simulink model "microarchi_router"  (R2015a)
settings: Solver=ode45  StartTime=0.0  StopTime=10.0  RelTol=1e-3
undefined symbols (not defined in the file or in its folder): des
(part 2 of 2)

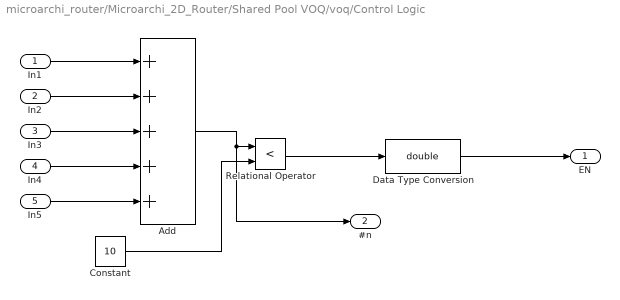
== system microarchi_router/Microarchi_2D_Router/Shared Pool VOQ/voq/Control Logic ==
  In1 : Inport
  In2 : Inport  Port=2
  In3 : Inport  Port=3
  In4 : Inport  Port=4
  In5 : Inport  Port=5
  Add : Sum  Inputs=+++++
  Constant : Constant  Value=10
  Data Type Conversion : DataTypeConversion  OutDataTypeStr=double
  Relational Operator : RelationalOperator  Operator=<
  EN : Outport  OutDataTypeStr=double
  #n : Outport  Port=2
  wires:
  In1/1 -> Add/1
  In2/1 -> Add/2
  In3/1 -> Add/3
  Constant/1 -> Relational Operator/2
  Add/1 -> #n/1, Relational Operator/1
  Relational Operator/1 -> Data Type Conversion/1
  Data Type Conversion/1 -> EN/1
  In4/1 -> Add/4
  In5/1 -> Add/5

== system microarchi_router/Microarchi_2D_Router/Shared Pool VOQ/voq/Release1 ==
  EN : Inport
  CLK : Inport  Port=2
  Enabled Gate6 : EnabledGate
  Out : PMIOPort  Port=1  Side=Right
  In : PMIOPort  Port=2  Side=Left
  wires:
  CLK/1 -> ?
  EN/1 -> Enabled Gate6/1
  connections:
  In/RConn1 -- Enabled Gate6/LConn1
  Enabled Gate6/RConn1 -- Out/RConn1

== system microarchi_router/Microarchi_2D_Router/Shared Pool VOQ/voq/Release2 ==
  EN : Inport
  CLK : Inport  Port=2
  Enabled Gate6 : EnabledGate
  Out : PMIOPort  Port=1  Side=Right
  In : PMIOPort  Port=2  Side=Left
  wires:
  EN/1 -> Enabled Gate6/1
  CLK/1 -> ?
  connections:
  Enabled Gate6/RConn1 -- Out/RConn1
  In/RConn1 -- Enabled Gate6/LConn1

== system microarchi_router/Microarchi_2D_Router/Shared Pool VOQ/voq/Release3 ==
  EN : Inport
  CLK : Inport  Port=2
  Enabled Gate6 : EnabledGate
  Out : PMIOPort  Port=1  Side=Right
  In : PMIOPort  Port=2  Side=Left
  wires:
  CLK/1 -> ?
  EN/1 -> Enabled Gate6/1
  connections:
  In/RConn1 -- Enabled Gate6/LConn1
  Enabled Gate6/RConn1 -- Out/RConn1

== system microarchi_router/Microarchi_2D_Router/Shared Pool VOQ/voq/Release4 ==
  EN : Inport
  CLK : Inport  Port=2
  Enabled Gate6 : EnabledGate
  Out : PMIOPort  Port=1  Side=Right
  In : PMIOPort  Port=2  Side=Left
  wires:
  EN/1 -> Enabled Gate6/1
  CLK/1 -> ?
  connections:
  Enabled Gate6/RConn1 -- Out/RConn1
  In/RConn1 -- Enabled Gate6/LConn1

== system microarchi_router/Microarchi_2D_Router/Shared Pool VOQ/voq/Release5 ==
  EN : Inport
  CLK : Inport  Port=2
  Enabled Gate6 : EnabledGate
  Out : PMIOPort  Port=1  Side=Right
  In : PMIOPort  Port=2  Side=Left
  wires:
  CLK/1 -> ?
  EN/1 -> Enabled Gate6/1
  connections:
  In/RConn1 -- Enabled Gate6/LConn1
  Enabled Gate6/RConn1 -- Out/RConn1

== system microarchi_router/Microarchi_2D_Router/Shared Pool VOQ1/voq/Clocked FIFO1 ==
  CLK : Inport
  FIFO Queue : FIFOQueue  Capacity=F  StatNumberInBlock=on
      settings: OutputPortMap=o1
  Release Gate : ReleaseGate  OpenGateUpon=Function call from port fcn
  Single Server : SingleServer  ServiceTime=0
  Input : PMIOPort  Port=1  Side=Left
  Output : PMIOPort  Port=2  Side=Right
  #n : Outport
  wires:
  CLK/1 -> Release Gate/1
  FIFO Queue/1 -> #n/1
  connections:
  FIFO Queue/LConn1 -- Input/RConn1
  Release Gate/RConn1 -- Output/RConn1
  Single Server/RConn1 -- Release Gate/LConn1
  FIFO Queue/RConn1 -- Single Server/LConn1

== system microarchi_router/Microarchi_2D_Router/Shared Pool VOQ1/voq/Clocked FIFO2 ==
  CLK : Inport
  FIFO Queue : FIFOQueue  Capacity=F  StatNumberInBlock=on
      settings: OutputPortMap=o1
  Release Gate : ReleaseGate  OpenGateUpon=Function call from port fcn
  Single Server : SingleServer  ServiceTime=0
  Input : PMIOPort  Port=1  Side=Left
  Output : PMIOPort  Port=2  Side=Right
  #n : Outport
  wires:
  FIFO Queue/1 -> #n/1
  CLK/1 -> Release Gate/1
  connections:
  FIFO Queue/RConn1 -- Single Server/LConn1
  Single Server/RConn1 -- Release Gate/LConn1
  Release Gate/RConn1 -- Output/RConn1
  FIFO Queue/LConn1 -- Input/RConn1

== system microarchi_router/Microarchi_2D_Router/Shared Pool VOQ1/voq/Clocked FIFO3 ==
  CLK : Inport
  FIFO Queue : FIFOQueue  Capacity=F  StatNumberInBlock=on
      settings: OutputPortMap=o1
  Release Gate : ReleaseGate  OpenGateUpon=Function call from port fcn
  Single Server : SingleServer  ServiceTime=0
  Input : PMIOPort  Port=1  Side=Left
  Output : PMIOPort  Port=2  Side=Right
  #n : Outport
  wires:
  CLK/1 -> Release Gate/1
  FIFO Queue/1 -> #n/1
  connections:
  FIFO Queue/LConn1 -- Input/RConn1
  Release Gate/RConn1 -- Output/RConn1
  Single Server/RConn1 -- Release Gate/LConn1
  FIFO Queue/RConn1 -- Single Server/LConn1

== system microarchi_router/Microarchi_2D_Router/Shared Pool VOQ1/voq/Clocked FIFO4 ==
  CLK : Inport
  FIFO Queue : FIFOQueue  Capacity=F  StatNumberInBlock=on
      settings: OutputPortMap=o1
  Release Gate : ReleaseGate  OpenGateUpon=Function call from port fcn
  Single Server : SingleServer  ServiceTime=0
  Input : PMIOPort  Port=1  Side=Left
  Output : PMIOPort  Port=2  Side=Right
  #n : Outport
  wires:
  FIFO Queue/1 -> #n/1
  CLK/1 -> Release Gate/1
  connections:
  FIFO Queue/RConn1 -- Single Server/LConn1
  Single Server/RConn1 -- Release Gate/LConn1
  Release Gate/RConn1 -- Output/RConn1
  FIFO Queue/LConn1 -- Input/RConn1

== system microarchi_router/Microarchi_2D_Router/Shared Pool VOQ1/voq/Clocked FIFO5 ==
  CLK : Inport
  FIFO Queue : FIFOQueue  Capacity=F  StatNumberInBlock=on
      settings: OutputPortMap=o1
  Release Gate : ReleaseGate  OpenGateUpon=Function call from port fcn
  Single Server : SingleServer  ServiceTime=0
  Input : PMIOPort  Port=1  Side=Left
  Output : PMIOPort  Port=2  Side=Right
  #n : Outport
  wires:
  CLK/1 -> Release Gate/1
  FIFO Queue/1 -> #n/1
  connections:
  FIFO Queue/LConn1 -- Input/RConn1
  Release Gate/RConn1 -- Output/RConn1
  Single Server/RConn1 -- Release Gate/LConn1
  FIFO Queue/RConn1 -- Single Server/LConn1

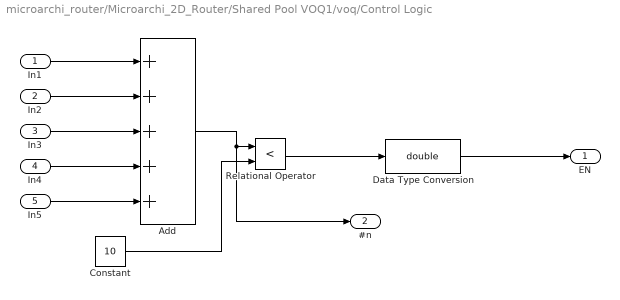
== system microarchi_router/Microarchi_2D_Router/Shared Pool VOQ1/voq/Control Logic ==
  In1 : Inport
  In2 : Inport  Port=2
  In3 : Inport  Port=3
  In4 : Inport  Port=4
  In5 : Inport  Port=5
  Add : Sum  Inputs=+++++
  Constant : Constant  Value=10
  Data Type Conversion : DataTypeConversion  OutDataTypeStr=double
  Relational Operator : RelationalOperator  Operator=<
  EN : Outport  OutDataTypeStr=double
  #n : Outport  Port=2
  wires:
  In5/1 -> Add/5
  In4/1 -> Add/4
  Data Type Conversion/1 -> EN/1
  Relational Operator/1 -> Data Type Conversion/1
  Add/1 -> Relational Operator/1, #n/1
  Constant/1 -> Relational Operator/2
  In3/1 -> Add/3
  In2/1 -> Add/2
  In1/1 -> Add/1

== system microarchi_router/Microarchi_2D_Router/Shared Pool VOQ1/voq/Release1 ==
  EN : Inport
  CLK : Inport  Port=2
  Enabled Gate6 : EnabledGate
  Out : PMIOPort  Port=1  Side=Right
  In : PMIOPort  Port=2  Side=Left
  wires:
  EN/1 -> Enabled Gate6/1
  CLK/1 -> ?
  connections:
  Enabled Gate6/RConn1 -- Out/RConn1
  In/RConn1 -- Enabled Gate6/LConn1

== system microarchi_router/Microarchi_2D_Router/Shared Pool VOQ1/voq/Release2 ==
  EN : Inport
  CLK : Inport  Port=2
  Enabled Gate6 : EnabledGate
  Out : PMIOPort  Port=1  Side=Right
  In : PMIOPort  Port=2  Side=Left
  wires:
  CLK/1 -> ?
  EN/1 -> Enabled Gate6/1
  connections:
  In/RConn1 -- Enabled Gate6/LConn1
  Enabled Gate6/RConn1 -- Out/RConn1

== system microarchi_router/Microarchi_2D_Router/Shared Pool VOQ1/voq/Release3 ==
  EN : Inport
  CLK : Inport  Port=2
  Enabled Gate6 : EnabledGate
  Out : PMIOPort  Port=1  Side=Right
  In : PMIOPort  Port=2  Side=Left
  wires:
  EN/1 -> Enabled Gate6/1
  CLK/1 -> ?
  connections:
  Enabled Gate6/RConn1 -- Out/RConn1
  In/RConn1 -- Enabled Gate6/LConn1

== system microarchi_router/Microarchi_2D_Router/Shared Pool VOQ1/voq/Release4 ==
  EN : Inport
  CLK : Inport  Port=2
  Enabled Gate6 : EnabledGate
  Out : PMIOPort  Port=1  Side=Right
  In : PMIOPort  Port=2  Side=Left
  wires:
  CLK/1 -> ?
  EN/1 -> Enabled Gate6/1
  connections:
  In/RConn1 -- Enabled Gate6/LConn1
  Enabled Gate6/RConn1 -- Out/RConn1

== system microarchi_router/Microarchi_2D_Router/Shared Pool VOQ1/voq/Release5 ==
  EN : Inport
  CLK : Inport  Port=2
  Enabled Gate6 : EnabledGate
  Out : PMIOPort  Port=1  Side=Right
  In : PMIOPort  Port=2  Side=Left
  wires:
  EN/1 -> Enabled Gate6/1
  CLK/1 -> ?
  connections:
  Enabled Gate6/RConn1 -- Out/RConn1
  In/RConn1 -- Enabled Gate6/LConn1

== system microarchi_router/Microarchi_2D_Router/Shared Pool VOQ2/voq/Clocked FIFO1 ==
  CLK : Inport
  FIFO Queue : FIFOQueue  Capacity=F  StatNumberInBlock=on
      settings: OutputPortMap=o1
  Release Gate : ReleaseGate  OpenGateUpon=Function call from port fcn
  Single Server : SingleServer  ServiceTime=0
  Input : PMIOPort  Port=1  Side=Left
  Output : PMIOPort  Port=2  Side=Right
  #n : Outport
  wires:
  FIFO Queue/1 -> #n/1
  CLK/1 -> Release Gate/1
  connections:
  FIFO Queue/RConn1 -- Single Server/LConn1
  Single Server/RConn1 -- Release Gate/LConn1
  Release Gate/RConn1 -- Output/RConn1
  FIFO Queue/LConn1 -- Input/RConn1

== system microarchi_router/Microarchi_2D_Router/Shared Pool VOQ2/voq/Clocked FIFO2 ==
  CLK : Inport
  FIFO Queue : FIFOQueue  Capacity=F  StatNumberInBlock=on
      settings: OutputPortMap=o1
  Release Gate : ReleaseGate  OpenGateUpon=Function call from port fcn
  Single Server : SingleServer  ServiceTime=0
  Input : PMIOPort  Port=1  Side=Left
  Output : PMIOPort  Port=2  Side=Right
  #n : Outport
  wires:
  CLK/1 -> Release Gate/1
  FIFO Queue/1 -> #n/1
  connections:
  FIFO Queue/LConn1 -- Input/RConn1
  Release Gate/RConn1 -- Output/RConn1
  Single Server/RConn1 -- Release Gate/LConn1
  FIFO Queue/RConn1 -- Single Server/LConn1

== system microarchi_router/Microarchi_2D_Router/Shared Pool VOQ2/voq/Clocked FIFO3 ==
  CLK : Inport
  FIFO Queue : FIFOQueue  Capacity=F  StatNumberInBlock=on
      settings: OutputPortMap=o1
  Release Gate : ReleaseGate  OpenGateUpon=Function call from port fcn
  Single Server : SingleServer  ServiceTime=0
  Input : PMIOPort  Port=1  Side=Left
  Output : PMIOPort  Port=2  Side=Right
  #n : Outport
  wires:
  FIFO Queue/1 -> #n/1
  CLK/1 -> Release Gate/1
  connections:
  FIFO Queue/RConn1 -- Single Server/LConn1
  Single Server/RConn1 -- Release Gate/LConn1
  Release Gate/RConn1 -- Output/RConn1
  FIFO Queue/LConn1 -- Input/RConn1

== system microarchi_router/Microarchi_2D_Router/Shared Pool VOQ2/voq/Clocked FIFO4 ==
  CLK : Inport
  FIFO Queue : FIFOQueue  Capacity=F  StatNumberInBlock=on
      settings: OutputPortMap=o1
  Release Gate : ReleaseGate  OpenGateUpon=Function call from port fcn
  Single Server : SingleServer  ServiceTime=0
  Input : PMIOPort  Port=1  Side=Left
  Output : PMIOPort  Port=2  Side=Right
  #n : Outport
  wires:
  CLK/1 -> Release Gate/1
  FIFO Queue/1 -> #n/1
  connections:
  FIFO Queue/LConn1 -- Input/RConn1
  Release Gate/RConn1 -- Output/RConn1
  Single Server/RConn1 -- Release Gate/LConn1
  FIFO Queue/RConn1 -- Single Server/LConn1

== system microarchi_router/Microarchi_2D_Router/Shared Pool VOQ2/voq/Clocked FIFO5 ==
  CLK : Inport
  FIFO Queue : FIFOQueue  Capacity=F  StatNumberInBlock=on
      settings: OutputPortMap=o1
  Release Gate : ReleaseGate  OpenGateUpon=Function call from port fcn
  Single Server : SingleServer  ServiceTime=0
  Input : PMIOPort  Port=1  Side=Left
  Output : PMIOPort  Port=2  Side=Right
  #n : Outport
  wires:
  FIFO Queue/1 -> #n/1
  CLK/1 -> Release Gate/1
  connections:
  FIFO Queue/RConn1 -- Single Server/LConn1
  Single Server/RConn1 -- Release Gate/LConn1
  Release Gate/RConn1 -- Output/RConn1
  FIFO Queue/LConn1 -- Input/RConn1

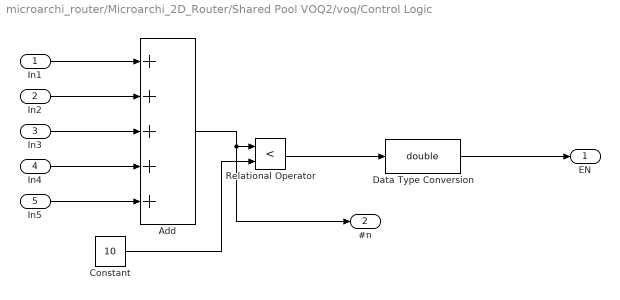
== system microarchi_router/Microarchi_2D_Router/Shared Pool VOQ2/voq/Control Logic ==
  In1 : Inport
  In2 : Inport  Port=2
  In3 : Inport  Port=3
  In4 : Inport  Port=4
  In5 : Inport  Port=5
  Add : Sum  Inputs=+++++
  Constant : Constant  Value=10
  Data Type Conversion : DataTypeConversion  OutDataTypeStr=double
  Relational Operator : RelationalOperator  Operator=<
  EN : Outport  OutDataTypeStr=double
  #n : Outport  Port=2
  wires:
  In1/1 -> Add/1
  In2/1 -> Add/2
  In3/1 -> Add/3
  Constant/1 -> Relational Operator/2
  Add/1 -> #n/1, Relational Operator/1
  Relational Operator/1 -> Data Type Conversion/1
  Data Type Conversion/1 -> EN/1
  In4/1 -> Add/4
  In5/1 -> Add/5

== system microarchi_router/Microarchi_2D_Router/Shared Pool VOQ2/voq/Release1 ==
  EN : Inport
  CLK : Inport  Port=2
  Enabled Gate6 : EnabledGate
  Out : PMIOPort  Port=1  Side=Right
  In : PMIOPort  Port=2  Side=Left
  wires:
  CLK/1 -> ?
  EN/1 -> Enabled Gate6/1
  connections:
  In/RConn1 -- Enabled Gate6/LConn1
  Enabled Gate6/RConn1 -- Out/RConn1

== system microarchi_router/Microarchi_2D_Router/Shared Pool VOQ2/voq/Release2 ==
  EN : Inport
  CLK : Inport  Port=2
  Enabled Gate6 : EnabledGate
  Out : PMIOPort  Port=1  Side=Right
  In : PMIOPort  Port=2  Side=Left
  wires:
  EN/1 -> Enabled Gate6/1
  CLK/1 -> ?
  connections:
  Enabled Gate6/RConn1 -- Out/RConn1
  In/RConn1 -- Enabled Gate6/LConn1

== system microarchi_router/Microarchi_2D_Router/Shared Pool VOQ2/voq/Release3 ==
  EN : Inport
  CLK : Inport  Port=2
  Enabled Gate6 : EnabledGate
  Out : PMIOPort  Port=1  Side=Right
  In : PMIOPort  Port=2  Side=Left
  wires:
  CLK/1 -> ?
  EN/1 -> Enabled Gate6/1
  connections:
  In/RConn1 -- Enabled Gate6/LConn1
  Enabled Gate6/RConn1 -- Out/RConn1

== system microarchi_router/Microarchi_2D_Router/Shared Pool VOQ2/voq/Release4 ==
  EN : Inport
  CLK : Inport  Port=2
  Enabled Gate6 : EnabledGate
  Out : PMIOPort  Port=1  Side=Right
  In : PMIOPort  Port=2  Side=Left
  wires:
  EN/1 -> Enabled Gate6/1
  CLK/1 -> ?
  connections:
  Enabled Gate6/RConn1 -- Out/RConn1
  In/RConn1 -- Enabled Gate6/LConn1

== system microarchi_router/Microarchi_2D_Router/Shared Pool VOQ2/voq/Release5 ==
  EN : Inport
  CLK : Inport  Port=2
  Enabled Gate6 : EnabledGate
  Out : PMIOPort  Port=1  Side=Right
  In : PMIOPort  Port=2  Side=Left
  wires:
  CLK/1 -> ?
  EN/1 -> Enabled Gate6/1
  connections:
  In/RConn1 -- Enabled Gate6/LConn1
  Enabled Gate6/RConn1 -- Out/RConn1

== system microarchi_router/Microarchi_2D_Router/Shared Pool VOQ3/voq/Clocked FIFO1 ==
  CLK : Inport
  FIFO Queue : FIFOQueue  Capacity=F  StatNumberInBlock=on
      settings: OutputPortMap=o1
  Release Gate : ReleaseGate  OpenGateUpon=Function call from port fcn
  Single Server : SingleServer  ServiceTime=0
  Input : PMIOPort  Port=1  Side=Left
  Output : PMIOPort  Port=2  Side=Right
  #n : Outport
  wires:
  CLK/1 -> Release Gate/1
  FIFO Queue/1 -> #n/1
  connections:
  FIFO Queue/LConn1 -- Input/RConn1
  Release Gate/RConn1 -- Output/RConn1
  Single Server/RConn1 -- Release Gate/LConn1
  FIFO Queue/RConn1 -- Single Server/LConn1

== system microarchi_router/Microarchi_2D_Router/Shared Pool VOQ3/voq/Clocked FIFO2 ==
  CLK : Inport
  FIFO Queue : FIFOQueue  Capacity=F  StatNumberInBlock=on
      settings: OutputPortMap=o1
  Release Gate : ReleaseGate  OpenGateUpon=Function call from port fcn
  Single Server : SingleServer  ServiceTime=0
  Input : PMIOPort  Port=1  Side=Left
  Output : PMIOPort  Port=2  Side=Right
  #n : Outport
  wires:
  FIFO Queue/1 -> #n/1
  CLK/1 -> Release Gate/1
  connections:
  FIFO Queue/RConn1 -- Single Server/LConn1
  Single Server/RConn1 -- Release Gate/LConn1
  Release Gate/RConn1 -- Output/RConn1
  FIFO Queue/LConn1 -- Input/RConn1

== system microarchi_router/Microarchi_2D_Router/Shared Pool VOQ3/voq/Clocked FIFO3 ==
  CLK : Inport
  FIFO Queue : FIFOQueue  Capacity=F  StatNumberInBlock=on
      settings: OutputPortMap=o1
  Release Gate : ReleaseGate  OpenGateUpon=Function call from port fcn
  Single Server : SingleServer  ServiceTime=0
  Input : PMIOPort  Port=1  Side=Left
  Output : PMIOPort  Port=2  Side=Right
  #n : Outport
  wires:
  CLK/1 -> Release Gate/1
  FIFO Queue/1 -> #n/1
  connections:
  FIFO Queue/LConn1 -- Input/RConn1
  Release Gate/RConn1 -- Output/RConn1
  Single Server/RConn1 -- Release Gate/LConn1
  FIFO Queue/RConn1 -- Single Server/LConn1

== system microarchi_router/Microarchi_2D_Router/Shared Pool VOQ3/voq/Clocked FIFO4 ==
  CLK : Inport
  FIFO Queue : FIFOQueue  Capacity=F  StatNumberInBlock=on
      settings: OutputPortMap=o1
  Release Gate : ReleaseGate  OpenGateUpon=Function call from port fcn
  Single Server : SingleServer  ServiceTime=0
  Input : PMIOPort  Port=1  Side=Left
  Output : PMIOPort  Port=2  Side=Right
  #n : Outport
  wires:
  FIFO Queue/1 -> #n/1
  CLK/1 -> Release Gate/1
  connections:
  FIFO Queue/RConn1 -- Single Server/LConn1
  Single Server/RConn1 -- Release Gate/LConn1
  Release Gate/RConn1 -- Output/RConn1
  FIFO Queue/LConn1 -- Input/RConn1

== system microarchi_router/Microarchi_2D_Router/Shared Pool VOQ3/voq/Clocked FIFO5 ==
  CLK : Inport
  FIFO Queue : FIFOQueue  Capacity=F  StatNumberInBlock=on
      settings: OutputPortMap=o1
  Release Gate : ReleaseGate  OpenGateUpon=Function call from port fcn
  Single Server : SingleServer  ServiceTime=0
  Input : PMIOPort  Port=1  Side=Left
  Output : PMIOPort  Port=2  Side=Right
  #n : Outport
  wires:
  CLK/1 -> Release Gate/1
  FIFO Queue/1 -> #n/1
  connections:
  FIFO Queue/LConn1 -- Input/RConn1
  Release Gate/RConn1 -- Output/RConn1
  Single Server/RConn1 -- Release Gate/LConn1
  FIFO Queue/RConn1 -- Single Server/LConn1

== system microarchi_router/Microarchi_2D_Router/Shared Pool VOQ3/voq/Control Logic ==
  In1 : Inport
  In2 : Inport  Port=2
  In3 : Inport  Port=3
  In4 : Inport  Port=4
  In5 : Inport  Port=5
  Add : Sum  Inputs=+++++
  Constant : Constant  Value=10
  Data Type Conversion : DataTypeConversion  OutDataTypeStr=double
  Relational Operator : RelationalOperator  Operator=<
  EN : Outport  OutDataTypeStr=double
  #n : Outport  Port=2
  wires:
  In5/1 -> Add/5
  In4/1 -> Add/4
  Data Type Conversion/1 -> EN/1
  Relational Operator/1 -> Data Type Conversion/1
  Add/1 -> Relational Operator/1, #n/1
  Constant/1 -> Relational Operator/2
  In3/1 -> Add/3
  In2/1 -> Add/2
  In1/1 -> Add/1

== system microarchi_router/Microarchi_2D_Router/Shared Pool VOQ3/voq/Release1 ==
  EN : Inport
  CLK : Inport  Port=2
  Enabled Gate6 : EnabledGate
  Out : PMIOPort  Port=1  Side=Right
  In : PMIOPort  Port=2  Side=Left
  wires:
  EN/1 -> Enabled Gate6/1
  CLK/1 -> ?
  connections:
  Enabled Gate6/RConn1 -- Out/RConn1
  In/RConn1 -- Enabled Gate6/LConn1

== system microarchi_router/Microarchi_2D_Router/Shared Pool VOQ3/voq/Release2 ==
  EN : Inport
  CLK : Inport  Port=2
  Enabled Gate6 : EnabledGate
  Out : PMIOPort  Port=1  Side=Right
  In : PMIOPort  Port=2  Side=Left
  wires:
  CLK/1 -> ?
  EN/1 -> Enabled Gate6/1
  connections:
  In/RConn1 -- Enabled Gate6/LConn1
  Enabled Gate6/RConn1 -- Out/RConn1

== system microarchi_router/Microarchi_2D_Router/Shared Pool VOQ3/voq/Release3 ==
  EN : Inport
  CLK : Inport  Port=2
  Enabled Gate6 : EnabledGate
  Out : PMIOPort  Port=1  Side=Right
  In : PMIOPort  Port=2  Side=Left
  wires:
  EN/1 -> Enabled Gate6/1
  CLK/1 -> ?
  connections:
  Enabled Gate6/RConn1 -- Out/RConn1
  In/RConn1 -- Enabled Gate6/LConn1

== system microarchi_router/Microarchi_2D_Router/Shared Pool VOQ3/voq/Release4 ==
  EN : Inport
  CLK : Inport  Port=2
  Enabled Gate6 : EnabledGate
  Out : PMIOPort  Port=1  Side=Right
  In : PMIOPort  Port=2  Side=Left
  wires:
  CLK/1 -> ?
  EN/1 -> Enabled Gate6/1
  connections:
  In/RConn1 -- Enabled Gate6/LConn1
  Enabled Gate6/RConn1 -- Out/RConn1

== system microarchi_router/Microarchi_2D_Router/Shared Pool VOQ3/voq/Release5 ==
  EN : Inport
  CLK : Inport  Port=2
  Enabled Gate6 : EnabledGate
  Out : PMIOPort  Port=1  Side=Right
  In : PMIOPort  Port=2  Side=Left
  wires:
  EN/1 -> Enabled Gate6/1
  CLK/1 -> ?
  connections:
  Enabled Gate6/RConn1 -- Out/RConn1
  In/RConn1 -- Enabled Gate6/LConn1

== system microarchi_router/Microarchi_2D_Router/Shared Pool VOQ4/voq/Clocked FIFO1 ==
  CLK : Inport
  FIFO Queue : FIFOQueue  Capacity=F  StatNumberInBlock=on
      settings: OutputPortMap=o1
  Release Gate : ReleaseGate  OpenGateUpon=Function call from port fcn
  Single Server : SingleServer  ServiceTime=0
  Input : PMIOPort  Port=1  Side=Left
  Output : PMIOPort  Port=2  Side=Right
  #n : Outport
  wires:
  FIFO Queue/1 -> #n/1
  CLK/1 -> Release Gate/1
  connections:
  FIFO Queue/RConn1 -- Single Server/LConn1
  Single Server/RConn1 -- Release Gate/LConn1
  Release Gate/RConn1 -- Output/RConn1
  FIFO Queue/LConn1 -- Input/RConn1

== system microarchi_router/Microarchi_2D_Router/Shared Pool VOQ4/voq/Clocked FIFO2 ==
  CLK : Inport
  FIFO Queue : FIFOQueue  Capacity=F  StatNumberInBlock=on
      settings: OutputPortMap=o1
  Release Gate : ReleaseGate  OpenGateUpon=Function call from port fcn
  Single Server : SingleServer  ServiceTime=0
  Input : PMIOPort  Port=1  Side=Left
  Output : PMIOPort  Port=2  Side=Right
  #n : Outport
  wires:
  CLK/1 -> Release Gate/1
  FIFO Queue/1 -> #n/1
  connections:
  FIFO Queue/LConn1 -- Input/RConn1
  Release Gate/RConn1 -- Output/RConn1
  Single Server/RConn1 -- Release Gate/LConn1
  FIFO Queue/RConn1 -- Single Server/LConn1

== system microarchi_router/Microarchi_2D_Router/Shared Pool VOQ4/voq/Clocked FIFO3 ==
  CLK : Inport
  FIFO Queue : FIFOQueue  Capacity=F  StatNumberInBlock=on
      settings: OutputPortMap=o1
  Release Gate : ReleaseGate  OpenGateUpon=Function call from port fcn
  Single Server : SingleServer  ServiceTime=0
  Input : PMIOPort  Port=1  Side=Left
  Output : PMIOPort  Port=2  Side=Right
  #n : Outport
  wires:
  FIFO Queue/1 -> #n/1
  CLK/1 -> Release Gate/1
  connections:
  FIFO Queue/RConn1 -- Single Server/LConn1
  Single Server/RConn1 -- Release Gate/LConn1
  Release Gate/RConn1 -- Output/RConn1
  FIFO Queue/LConn1 -- Input/RConn1

== system microarchi_router/Microarchi_2D_Router/Shared Pool VOQ4/voq/Clocked FIFO4 ==
  CLK : Inport
  FIFO Queue : FIFOQueue  Capacity=F  StatNumberInBlock=on
      settings: OutputPortMap=o1
  Release Gate : ReleaseGate  OpenGateUpon=Function call from port fcn
  Single Server : SingleServer  ServiceTime=0
  Input : PMIOPort  Port=1  Side=Left
  Output : PMIOPort  Port=2  Side=Right
  #n : Outport
  wires:
  CLK/1 -> Release Gate/1
  FIFO Queue/1 -> #n/1
  connections:
  FIFO Queue/LConn1 -- Input/RConn1
  Release Gate/RConn1 -- Output/RConn1
  Single Server/RConn1 -- Release Gate/LConn1
  FIFO Queue/RConn1 -- Single Server/LConn1

== system microarchi_router/Microarchi_2D_Router/Shared Pool VOQ4/voq/Clocked FIFO5 ==
  CLK : Inport
  FIFO Queue : FIFOQueue  Capacity=F  StatNumberInBlock=on
      settings: OutputPortMap=o1
  Release Gate : ReleaseGate  OpenGateUpon=Function call from port fcn
  Single Server : SingleServer  ServiceTime=0
  Input : PMIOPort  Port=1  Side=Left
  Output : PMIOPort  Port=2  Side=Right
  #n : Outport
  wires:
  FIFO Queue/1 -> #n/1
  CLK/1 -> Release Gate/1
  connections:
  FIFO Queue/RConn1 -- Single Server/LConn1
  Single Server/RConn1 -- Release Gate/LConn1
  Release Gate/RConn1 -- Output/RConn1
  FIFO Queue/LConn1 -- Input/RConn1

== system microarchi_router/Microarchi_2D_Router/Shared Pool VOQ4/voq/Control Logic ==
  In1 : Inport
  In2 : Inport  Port=2
  In3 : Inport  Port=3
  In4 : Inport  Port=4
  In5 : Inport  Port=5
  Add : Sum  Inputs=+++++
  Constant : Constant  Value=10
  Data Type Conversion : DataTypeConversion  OutDataTypeStr=double
  Relational Operator : RelationalOperator  Operator=<
  EN : Outport  OutDataTypeStr=double
  #n : Outport  Port=2
  wires:
  In1/1 -> Add/1
  In2/1 -> Add/2
  In3/1 -> Add/3
  Constant/1 -> Relational Operator/2
  Add/1 -> #n/1, Relational Operator/1
  Relational Operator/1 -> Data Type Conversion/1
  Data Type Conversion/1 -> EN/1
  In4/1 -> Add/4
  In5/1 -> Add/5

== system microarchi_router/Microarchi_2D_Router/Shared Pool VOQ4/voq/Release1 ==
  EN : Inport
  CLK : Inport  Port=2
  Enabled Gate6 : EnabledGate
  Out : PMIOPort  Port=1  Side=Right
  In : PMIOPort  Port=2  Side=Left
  wires:
  CLK/1 -> ?
  EN/1 -> Enabled Gate6/1
  connections:
  In/RConn1 -- Enabled Gate6/LConn1
  Enabled Gate6/RConn1 -- Out/RConn1

== system microarchi_router/Microarchi_2D_Router/Shared Pool VOQ4/voq/Release2 ==
  EN : Inport
  CLK : Inport  Port=2
  Enabled Gate6 : EnabledGate
  Out : PMIOPort  Port=1  Side=Right
  In : PMIOPort  Port=2  Side=Left
  wires:
  EN/1 -> Enabled Gate6/1
  CLK/1 -> ?
  connections:
  Enabled Gate6/RConn1 -- Out/RConn1
  In/RConn1 -- Enabled Gate6/LConn1

== system microarchi_router/Microarchi_2D_Router/Shared Pool VOQ4/voq/Release3 ==
  EN : Inport
  CLK : Inport  Port=2
  Enabled Gate6 : EnabledGate
  Out : PMIOPort  Port=1  Side=Right
  In : PMIOPort  Port=2  Side=Left
  wires:
  CLK/1 -> ?
  EN/1 -> Enabled Gate6/1
  connections:
  In/RConn1 -- Enabled Gate6/LConn1
  Enabled Gate6/RConn1 -- Out/RConn1

== system microarchi_router/Microarchi_2D_Router/Shared Pool VOQ4/voq/Release4 ==
  EN : Inport
  CLK : Inport  Port=2
  Enabled Gate6 : EnabledGate
  Out : PMIOPort  Port=1  Side=Right
  In : PMIOPort  Port=2  Side=Left
  wires:
  EN/1 -> Enabled Gate6/1
  CLK/1 -> ?
  connections:
  Enabled Gate6/RConn1 -- Out/RConn1
  In/RConn1 -- Enabled Gate6/LConn1

== system microarchi_router/Microarchi_2D_Router/Shared Pool VOQ4/voq/Release5 ==
  EN : Inport
  CLK : Inport  Port=2
  Enabled Gate6 : EnabledGate
  Out : PMIOPort  Port=1  Side=Right
  In : PMIOPort  Port=2  Side=Left
  wires:
  CLK/1 -> ?
  EN/1 -> Enabled Gate6/1
  connections:
  In/RConn1 -- Enabled Gate6/LConn1
  Enabled Gate6/RConn1 -- Out/RConn1

== matlab function microarchi_router/Microarchi_2D_Router/Route XY/Attribute Function/MATLAB Function ==
  data: DST_X input; DST_Y input; out_RT output; IME_X input; IME_Y input
  events: trigger input FUNCTION_CALL_EVENT
function out_RT  = fcn(DST_X,DST_Y, IME_X, IME_Y)
%FCN    Access and modify attributes with MATLAB 
% 
% Input arguments must match the attribute names.
% Output arguments must be out_<AttributeName>,
% e.g., out_ServiceTime where ServiceTime is the attribute name.
% 
% The output attribute will be created if it is not present.
%

North = 1;
South = 2;
West = 3;
East = 4;
NI = 5;

xi =IME_X;
yi =IME_Y;



x = DST_X;
y = DST_Y;


if (xi ~= x),
    if (xi > x),
        out_RT = West;
    else
        out_RT = East;
    end
elseif (yi ~= y),
    if (yi > y),
        out_RT = North;
    else
        out_RT = South;
    end

else
    out_RT = NI;
end

== matlab function microarchi_router/Microarchi_2D_Router/Route XY1/Attribute Function/MATLAB Function ==
  data: DST_X input; DST_Y input; out_RT output; IME_X input; IME_Y input
  events: trigger input FUNCTION_CALL_EVENT
function out_RT  = fcn(DST_X,DST_Y, IME_X, IME_Y)
%FCN    Access and modify attributes with MATLAB 
% 
% Input arguments must match the attribute names.
% Output arguments must be out_<AttributeName>,
% e.g., out_ServiceTime where ServiceTime is the attribute name.
% 
% The output attribute will be created if it is not present.
%

North = 1;
South = 2;
West = 3;
East = 4;
NI = 5;

xi =IME_X;
yi =IME_Y;



x = DST_X;
y = DST_Y;


if (xi ~= x),
    if (xi > x),
        out_RT = West;
    else
        out_RT = East;
    end
elseif (yi ~= y),
    if (yi > y),
        out_RT = North;
    else
        out_RT = South;
    end

else
    out_RT = NI;
end

== matlab function microarchi_router/Microarchi_2D_Router/Route XY2/Attribute Function/MATLAB Function ==
  data: DST_X input; DST_Y input; out_RT output; IME_X input; IME_Y input
  events: trigger input FUNCTION_CALL_EVENT
function out_RT  = fcn(DST_X,DST_Y, IME_X, IME_Y)
%FCN    Access and modify attributes with MATLAB 
% 
% Input arguments must match the attribute names.
% Output arguments must be out_<AttributeName>,
% e.g., out_ServiceTime where ServiceTime is the attribute name.
% 
% The output attribute will be created if it is not present.
%

North = 1;
South = 2;
West = 3;
East = 4;
NI = 5;

xi =IME_X;
yi =IME_Y;



x = DST_X;
y = DST_Y;


if (xi ~= x),
    if (xi > x),
        out_RT = West;
    else
        out_RT = East;
    end
elseif (yi ~= y),
    if (yi > y),
        out_RT = North;
    else
        out_RT = South;
    end

else
    out_RT = NI;
end

== matlab function microarchi_router/Microarchi_2D_Router/Route XY3/Attribute Function/MATLAB Function ==
  data: DST_X input; DST_Y input; out_RT output; IME_X input; IME_Y input
  events: trigger input FUNCTION_CALL_EVENT
function out_RT  = fcn(DST_X,DST_Y, IME_X, IME_Y)
%FCN    Access and modify attributes with MATLAB 
% 
% Input arguments must match the attribute names.
% Output arguments must be out_<AttributeName>,
% e.g., out_ServiceTime where ServiceTime is the attribute name.
% 
% The output attribute will be created if it is not present.
%

North = 1;
South = 2;
West = 3;
East = 4;
NI = 5;

xi =IME_X;
yi =IME_Y;



x = DST_X;
y = DST_Y;


if (xi ~= x),
    if (xi > x),
        out_RT = West;
    else
        out_RT = East;
    end
elseif (yi ~= y),
    if (yi > y),
        out_RT = North;
    else
        out_RT = South;
    end

else
    out_RT = NI;
end

== matlab function microarchi_router/Microarchi_2D_Router/Arbiter/MATLAB Function ==
  data: v1 input; p1 output; v2 input; v3 input; v4 input; p2 output; p3 output; p4 output; v5 input; p5 output
function [p1,p2,p3,p4,p5] = fcn(v1,v2,v3,v4,v5)
%#codegen
%keyboard
[~,s1] = sort(v1,'descend');
[~,s2] = sort(v2,'descend');
[~,s3] = sort(v3,'descend');
[~,s4] = sort(v4,'descend');


V = [v1 v2 v3 v4];
S = [s1 s2 s3 s4]+1;

[~,k] = find(V(1,:)~=0);
[~,l] = find(V(1,:)==0);


P = zeros(1,4);

P(k) = S(2,k);

for i=3:5,
    if (length(unique(P))~=length(P)),
        
    else 
        break;
    end
end


P = randperm(5);

p1 = P(1);
p2 = P(2);
p3 = P(3);
p4 = P(4);
p5 = P(5);

== matlab function microarchi_router/Microarchi_2D_Router/Route XY4/Attribute Function/MATLAB Function ==
  data: DST_X input; DST_Y input; out_RT output; IME_X input; IME_Y input
  events: trigger input FUNCTION_CALL_EVENT
function out_RT  = fcn(DST_X,DST_Y, IME_X, IME_Y)
%FCN    Access and modify attributes with MATLAB 
% 
% Input arguments must match the attribute names.
% Output arguments must be out_<AttributeName>,
% e.g., out_ServiceTime where ServiceTime is the attribute name.
% 
% The output attribute will be created if it is not present.
%

North = 1;
South = 2;
West = 3;
East = 4;
NI = 5;

xi =IME_X;
yi =IME_Y;



x = DST_X;
y = DST_Y;


if (xi ~= x),
    if (xi > x),
        out_RT = West;
    else
        out_RT = East;
    end
elseif (yi ~= y),
    if (yi > y),
        out_RT = North;
    else
        out_RT = South;
    end

else
    out_RT = NI;
end
